simulink model "AMR_VehicleSpeedReadout"  (R2024a)
settings: Solver=FixedStepDiscrete  StartTime=0.0  StopTime=inf  FixedStep=10e-3  RelTol=1e-3
values from neighbouring files (symbols this model uses):
  car_wheel_base = 877.0    [configuration_dictionary.sldd]
  gearbox_ratio = 40.61    [configuration_dictionary.sldd]
  wheel_diameter = 360.0    [configuration_dictionary.sldd]
settings Model: DataDictionary=configuration_dictionary.sldd  Creator=matlab.cut  LastModifiedBy=rodri
settings SolverCC: ConcurrentTasks=on  PositivePriorityOrder=on
settings OptimizationCC: BlockReduction=off  DefaultParameterBehavior=Inlined  OptimizeBlockIOStorage=off
settings DebuggingCC: TasksWithSamePriorityMsg=none
settings HardwareCC: ProdBitPerLong=64  ProdLongLongMode=on  ProdHWDeviceType=Intel->x86-64 (Linux 64)
settings SFSimCC: MATLABDynamicMemAlloc=off
settings RTWCC: Description=Speedgoat Real-Time Target Machine  SystemTargetFile=speedgoat.tlc  TemplateMakefile=slrealtime_default_tmf  Toolchain=Simulink Real-Time Toolchain  BuildConfiguration=Faster Runs  CodeExecutionProfiling=on  TargetLang=C++  GPUComputeCapability=3.5
settings SimulinkRealTimeTargetCC: InstructionSetFMA=off  LogToMDFFile=off

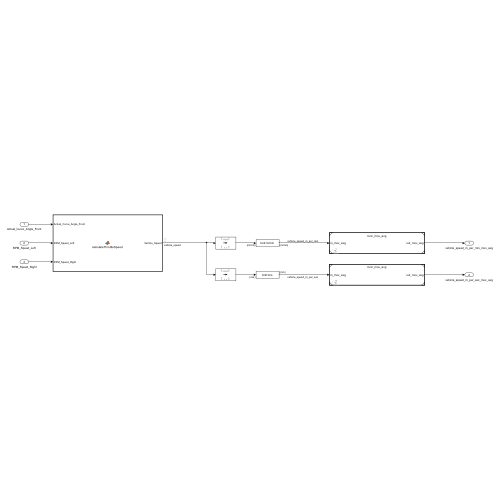
[thumbnail: Simulink's stored preview of the top-level diagram]
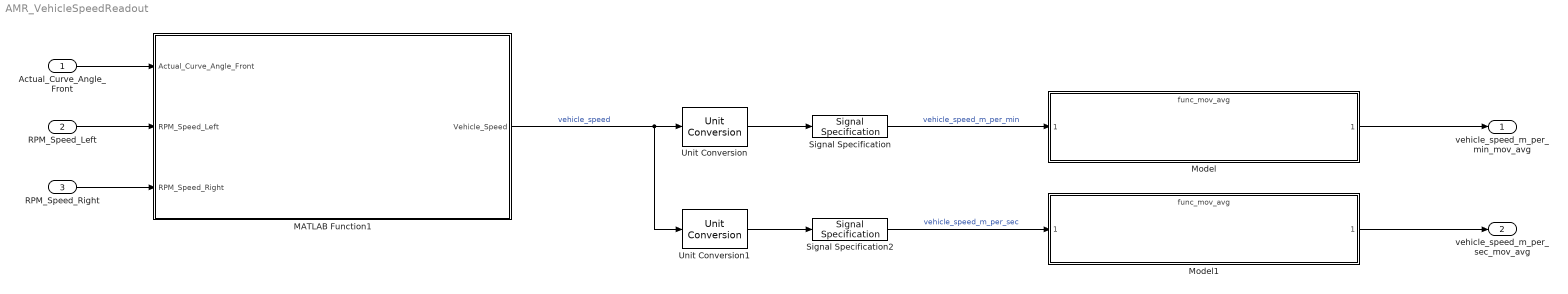
== system AMR_VehicleSpeedReadout ==
  Actual_Curve_Angle_Front : Inport
  RPM_Speed_Left : Inport  Port=2
  RPM_Speed_Right : Inport  Port=3
  MATLAB Function1 : MATLAB Function  TreatAsAtomicUnit=on
  Model : ModelReference  ModelNameDialog=func_mov_avg.slx  SimulationMode=Normal  ModelReferenceVersion=1.7
  Model1 : ModelReference  ModelNameDialog=func_mov_avg.slx  SimulationMode=Normal  ModelReferenceVersion=1.7
  Signal Specification : SignalSpecification  Unit=m/min
  Signal Specification2 : SignalSpecification  Unit=m/s
  Unit Conversion : UnitConversion  OutputType=Inherit: Inherit via back propagation
  Unit Conversion1 : UnitConversion  OutputType=Inherit: Inherit via back propagation
  vehicle_speed_m_per_min_mov_avg : Outport
  vehicle_speed_m_per_sec_mov_avg : Outport  Port=2
  wires:
  MATLAB Function1/1(Vehicle_Speed) -> Unit Conversion1/1, Unit Conversion/1  "vehicle_speed"
  RPM_Speed_Right/1 -> MATLAB Function1/3(RPM_Speed_Right)
  RPM_Speed_Left/1 -> MATLAB Function1/2(RPM_Speed_Left)
  Actual_Curve_Angle_Front/1 -> MATLAB Function1/1(Actual_Curve_Angle_Front)
  Unit Conversion/1 -> Signal Specification/1
  Unit Conversion1/1 -> Signal Specification2/1
  Signal Specification/1 -> Model/1  "vehicle_speed_m_per_min"
  Model/1 -> vehicle_speed_m_per_min_mov_avg/1
  Signal Specification2/1 -> Model1/1  "vehicle_speed_m_per_sec"
  Model1/1 -> vehicle_speed_m_per_sec_mov_avg/1

== matlab function AMR_VehicleSpeedReadout/MATLAB Function1 ==
  data: Actual_Curve_Angle_Front input; Vehicle_Speed output; RPM_Speed_Left input; RPM_Speed_Right input; car_wheel_base parameter; wheel_diameter parameter; gearbox_ratio parameter
function Vehicle_Speed = calculateThrottleSpeed(Actual_Curve_Angle_Front, RPM_Speed_Left, RPM_Speed_Right, car_wheel_base, wheel_diameter, gearbox_ratio)

    PAR_Wheel_Base = car_wheel_base;
    PAR_Drive_Wheel_Offset = PAR_Wheel_Base/2;

    if Actual_Curve_Angle_Front == 0
        Mean_Motor_Speed = (RPM_Speed_Left + RPM_Speed_Right) / 2;
    elseif Actual_Curve_Angle_Front < 0
        Radius_C = PAR_Wheel_Base / tan(deg2rad(abs(Actual_Curve_Angle_Front)));
        Mean_Motor_Speed = (RPM_Speed_Left * Radius_C + RPM_Speed_Right * (Radius_C - PAR_Drive_Wheel_Offset)) / (2 * Radius_C - PAR_Drive_Wheel_Offset);
    else
        Radius_C = PAR_Wheel_Base / tan(deg2rad(abs(Actual_Curve_Angle_Front)));
        Mean_Motor_Speed = (RPM_Speed_Left * Radius_C + RPM_Speed_Right * (Radius_C + PAR_Drive_Wheel_Offset)) / (2 * Radius_C + PAR_Drive_Wheel_Offset);
    end
    
    Vehicle_Speed = Mean_Motor_Speed * wheel_diameter * pi / gearbox_ratio;

end
